simulink model "FreqAdaptiveFFT"  (R2018a)
settings: Solver=ode8  StartTime=0.0  StopTime=Ttot  FixedStep=Ts  RelTol=1e-3
values from neighbouring files (symbols this model uses):
  Ts = Ts_control / 60    (= 9.25925925926e-07)    [Equivalency_Script.m]    (also in FreqAdaptiveFFT_Script.m; FreqAdaptive_Script.m; ShortPulse_Script.m)
  Ts_control = 1/(300*Fn)    (= 5.55555555556e-05)    [Equivalency_Script.m]    (also in FreqAdaptiveFFT_Script.m; FreqAdaptive_Script.m; ShortPulse_Script.m)
libraries: powerlib x1
settings Model: SimulationMode=accelerator  Creator=daniemot  LastModifiedBy=daniemot
settings SolverCC: AutoInsertRateTranBlk=on
settings DataIOCC: ExternalInput=getinputstruct(WN_50mF_op_snapshot1)  InitialState=getstatestruct(WN_50mF_op_snapshot1)  SaveFinalState=on  SaveFormat=StructureWithTime  SaveOutput=off  SignalLogging=off  DSMLogging=off  SaveTime=off
settings DebuggingCC: ReadBeforeWriteMsg=DisableAll  WriteAfterWriteMsg=DisableAll  WriteAfterReadMsg=DisableAll  MultiTaskDSMMsg=none  UnconnectedInputMsg=none  UnconnectedOutputMsg=none  UnconnectedLineMsg=none
settings ModelReferenceCC: UpdateModelReferenceTargets=IfOutOfDate
settings SFSimCC: SFSimEcho=off

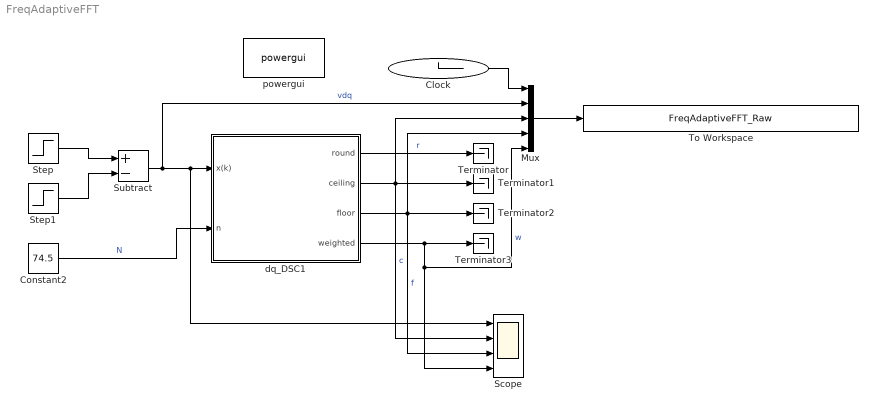
== system FreqAdaptiveFFT ==
  Clock : Clock
  Constant2 : Constant  Value=74.5
  Mux : Mux  Inputs=5
  Scope : Scope  NumInputPorts=4
  Step : Step  Time=0  SampleTime=0
  Step1 : Step  Time=Ts_control  SampleTime=0
  Subtract : Sum  Inputs=+-
  Terminator{,1..3} (4 alike) : Terminator
  To Workspace : ToWorkspace  VariableName=FreqAdaptiveFFT_Raw  SampleTime=Ts_control
      settings: Save2DSignal=2-D array (concatenate along first dimension)
  dq_DSC1 : Subsystem  TreatAsAtomicUnit=on  SystemSampleTime=Ts  mask{Ts=Ts_control, nmax=200}
      mask prompts: Ts "Sample times [s]"; nmax "Maximum delay nmax:"
      mask Display: fprintf('y(k)=0.5(x(k)+x(k-n))');
  powergui : powerlib/powergui  Priority=1  SimulationMode=Discrete  SampleTime=Ts  frequency=60  Iterations=50  frequencyindice=0  Pbase=100e6  ErrMax=1e-4  UnitsV=kV  UnitsW=MW  buscounter=0  FunctionMessages=off  echomessages=off  EnableUseOfTLC=off  CurrentSourceSwitches=off  DisableSnubberDevices=off  DisableRonSwitches=off  DisableVfSwitches=off  DisplayEquations=off  SolverType=Tustin/Backward Euler (TBE)  Interpol=off  ExternalGateDelay=off  methode=off  Ts=100  x0status=blocks  SPID=off  SwTol=0  HookPort=off  RestoreLinks=warning  ResistiveCurrentMeasurement=off  Frange=[60:1:1600]  Ylog=on  Xlog=on  ShowGrid=on  save=off  variable=ZData  structure=0  ZoomFFT=off  StartTime=0.0  cycles=1  DisplayStyle=1  fundamental=60  FreqAxis=off  MaxFrequency=1000  frequencyindicesteady=1  RmsSteady=1  display=off
  wires:
  Subtract/1 -> Mux/2, dq_DSC1/1(x(k)), Scope/1  "vdq"
  Constant2/1 -> dq_DSC1/2(n)  "N"
  dq_DSC1/1(round) -> Terminator/1  "r"
  dq_DSC1/2(ceiling) -> Mux/3, Scope/2, Terminator1/1  "c"
  dq_DSC1/3(floor) -> Mux/4, Scope/3, Terminator2/1  "f"
  dq_DSC1/4(weighted) -> Mux/5, Scope/4, Terminator3/1  "w"
  Step/1 -> Subtract/1
  Step1/1 -> Subtract/2
  Mux/1 -> To Workspace/1
  Clock/1 -> Mux/1

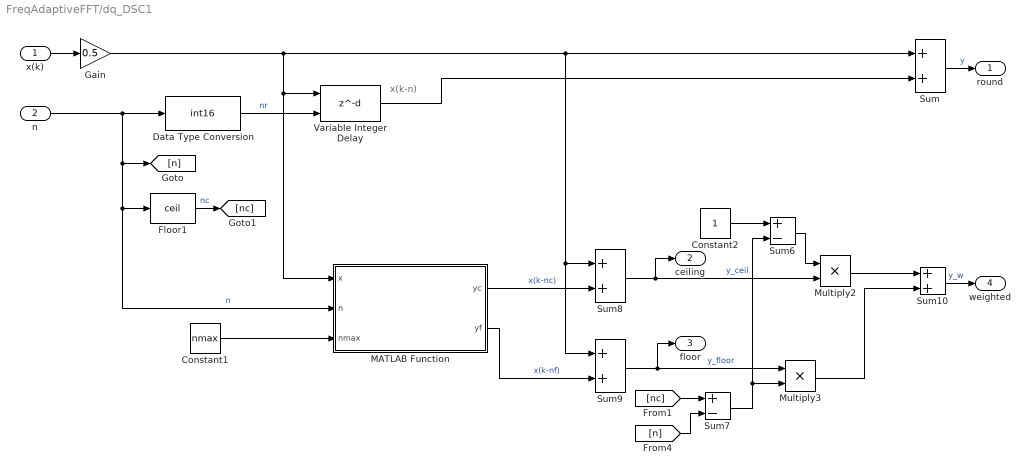
== system FreqAdaptiveFFT/dq_DSC1 ==
  note: x(k-n)
  x(k) : Inport
  n : Inport  Port=2
  Constant1 : Constant  Value=nmax
  Constant2 : Constant
  Data Type Conversion : DataTypeConversion  OutDataTypeStr=int16  RndMeth=Round  SaturateOnIntegerOverflow=on
  Floor1 : Rounding  Operator=ceil
  Gain : Gain  Gain=0.5
  MATLAB Function : MATLAB Function  TreatAsAtomicUnit=on  SystemSampleTime=Ts_control
  Multiply2 : Product
  Multiply3 : Product
  Sum{,8..10} (4 alike) : Sum
  Sum6 : Sum  Inputs=+-
  Sum7 : Sum  Inputs=+-
  Variable Integer Delay : Delay  DelayLengthSource=Input port  DelayLength=200  DelayLengthUpperLimit=nmax  SampleTime=Ts
      settings: InputPortMap=u0,p1
  round : Outport
  ceiling : Outport  Port=2
  floor : Outport  Port=3
  weighted : Outport  Port=4
  wires:
  Sum/1 -> round/1  "y"
  Data Type Conversion/1 -> Variable Integer Delay/2  "nr"
  Floor1/1 -> [nc]  "nc"
  Variable Integer Delay/1 -> Sum/2
  x(k)/1 -> Gain/1
  n/1 -> Data Type Conversion/1, Floor1/1, MATLAB Function/2(n), [n]  "n"
  Constant1/1 -> MATLAB Function/3(nmax)
  [n] -> Sum7/2
  MATLAB Function/1(yc) -> Sum8/2  "x(k-nc)"
  Sum7/1 -> Sum6/2, Multiply3/2
  Constant2/1 -> Sum6/1
  Sum6/1 -> Multiply2/1
  MATLAB Function/2(yf) -> Sum9/2  "x(k-nf)"
  Sum8/1 -> ceiling/1, Multiply2/2  "y_ceil"
  Sum9/1 -> floor/1, Multiply3/1  "y_floor"
  Sum10/1 -> weighted/1  "y_w"
  Gain/1 -> Sum/1, Sum9/1, Sum8/1, Variable Integer Delay/1, MATLAB Function/1(x)
  Multiply3/1 -> Sum10/2
  [nc] -> Sum7/1
  Multiply2/1 -> Sum10/1

== matlab function FreqAdaptiveFFT/dq_DSC1/MATLAB Function ==
  data: x input; yc output; n input; yf output; nmax input
function [yc,    yf]  = CircBuff_Delay_CeilFloor(x, n, nmax)
%% %%%%%%%%%%%%%%%%%%%%%%%%%%%%%%%%%%%%%%%%%%%%%%%%%%%%%%%%%%%%%%%%%%%%%%%%
% Circular Buffer 
% By: Mota
% Revision history:
%       2021-07-16: first release
%
%%Interface  
%   Inputs
%       x : scalar
%       n : delay in samples (float, ideal delay is time was continuous)
%       nmax : max size of circular buffer, ONLY used in FIRST CYCLE
%
%   Output
%       yc = x(k - ceil(n))
%       yf = x(k - floor(n))
% 

persistent CB       % circular buffer, created with zeros in first cycle
persistent ins_p    % insertion pointer, integer, zero -> Nmax-1
persistent Nmax     % Buffer lenght, updated ONLY in FIRST CYCLE


%% Initialization of persistent variables
if isempty(Nmax)
    if nmax < 5     % Hardcoded minimum lenght of buffer (arbitrary)
        Nmax = 5;
    else 
        Nmax = round(nmax); % No limit for maximum lenght of buffer 
    end
    
    CB = zeros(Nmax, 1);    % circular buffer
                            % Nmax lines x 2 columns 
                            % Column 1: ceiling 
                            % Column 2: floor
    
    ins_p = 0;      % Insertion pointer initialization
    
end

%% %%%%%%%%%%%%%%%%%%%%%%%%%%%%%%%%%%%%%%%%%%%%%%%%%%%%%%%%%%%%%%%%%%%%%%
% Insertion of current values
%%%%%%%%%%%%%%%%%%%%%%%%%%%%%%%%%%%%%%%%%%%%%%%%%%%%%%%%%%%%%%%%%%%%%%%%%
CB(ins_p + 1) = x;    

%% %%%%%%%%%%%%%%%%%%%%%%%%%%%%%%%%%%%%%%%%%%%%%%%%%%%%%%%%%%%%%%%%%%%%%%
% Retrieval pointer calculation
%   Be careful with confusion of indices
%       Matlab index for array:     1, 2,... Nmax
%       Insertion pointer values:   0, 1,... Nmax - 1
%%%%%%%%%%%%%%%%%%%%%%%%%%%%%%%%%%%%%%%%%%%%%%%%%%%%%%%%%%%%%%%%%%%%%%%%%
if n >= 1       
    if n <= Nmax - 1    % if 1 >= n >= Nmax - 1 
                        % n cannot be equal to Nmax, or else the retrieval
                        % pointers retreat back to the the insertion
                        % pointer.
                                
        p_r_c = mod(ins_p - ceil(n), Nmax); % ceiling retrieval pointer
        p_r_f = mod(ins_p - floor(n), Nmax); % floor retrieval pointer
    
    else
        % The maximum delay is Nmax - 1
        p_r_c = mod(ins_p - Nmax - 1, Nmax);
        p_r_f = mod(ins_p - Nmax - 1, Nmax);
    end
else
    % Minimul delay is zero
    p_r_c = ins_p;
    p_r_f = ins_p;
end
    
%% %%%%%%%%%%%%%%%%%%%%%%%%%%%%%%%%%%%%%%%%%%%%%%%%%%%%%%%%%%%%%%%%%%%%%%
% Temporary variables with retrieved values
%   CB indexes: 1, 2, ... Nmax
%%%%%%%%%%%%%%%%%%%%%%%%%%%%%%%%%%%%%%%%%%%%%%%%%%%%%%%%%%%%%%%%%%%%%%%%%
col1_c = CB(p_r_c + 1); 
col1_f = CB(p_r_f + 1);


%% %%%%%%%%%%%%%%%%%%%%%%%%%%%%%%%%%%%%%%%%%%%%%%%%%%%%%%%%%%%%%%%%%%%%%%
% Outputs vectors
%%%%%%%%%%%%%%%%%%%%%%%%%%%%%%%%%%%%%%%%%%%%%%%%%%%%%%%%%%%%%%%%%%%%%%%%%
yc = col1_c;
yf = col1_f;

%% %%%%%%%%%%%%%%%%%%%%%%%%%%%%%%%%%%%%%%%%%%%%%%%%%%%%%%%%%%%%%%%%%%%%%%
% Update Outputs vectors
%%%%%%%%%%%%%%%%%%%%%%%%%%%%%%%%%%%%%%%%%%%%%%%%%%%%%%%%%%%%%%%%%%%%%%%%%
ins_p = mod(ins_p + 1, Nmax);
